simulink model "Prosthesis"  (R2014a)
settings: Solver=ode15s  StartTime=0.0  StopTime=20  MaxStep=.01  RelTol=1e-4  AbsTol=1e-5
InitFcn:
  | RphiKnee0 = 0*pi/180;
  | RphiAnkle0 = 0;
  | prostheticParams
StartFcn:
  | tic;
StopFcn:
  | toc
values from neighbouring files (symbols this model uses):
  ankleBackDriveGain = 0.8    [prostheticParams.m]
  ankleDgain = 0.001    [prostheticParams.m]
  ankleFilterPID = 100    [prostheticParams.m]
  ankleFilterSEA = 100    [prostheticParams.m]
  ankleGearEff = 1.00    (= 1)    [prostheticParams.m]
  ankleGearRatio = 50    [prostheticParams.m]
  ankleIgain = 0.00    (= 0)    [prostheticParams.m]
  ankleInitialAngle = -RphiAnkle0    [prostheticParams.m]
  ankleInputMass = 2329.69    [prostheticParams.m]
  ankleParallelSpringDamping = ankleParallelSpringStiffness/200    (= 0.95)    [prostheticParams.m]
  ankleParallelSpringOffset = 0    [prostheticParams.m]
  ankleParallelSpringStiffness = 190    [prostheticParams.m]
  anklePgain = 0.01    [prostheticParams.m]
  ankleSEADamping = ankleSEAStiffness/100    (= 15)    [prostheticParams.m]
  ankleSEAStiffness = 1500    [prostheticParams.m]
  ankleTendonMass = 36.26    [prostheticParams.m]
  footMassp = 690.10    (= 690.1)    [prostheticParams.m]
  FourBarL1 = 0.080    (= 0.08)    [prostheticParams.m]
  FourBarL3 = 0.0826238    [prostheticParams.m]
  kneeBackDriveGain = 0.8    [prostheticParams.m]
  kneeDgain = 0.001    [prostheticParams.m]
  kneeFilterPID = 100    [prostheticParams.m]
  kneeFilterSEA = 100    [prostheticParams.m]
  kneeGearEff = 1.00    (= 1)    [prostheticParams.m]
  kneeGearRatio = 50    [prostheticParams.m]
  kneeIgain = 0.00    (= 0)    [prostheticParams.m]
  kneeInitialAngle = -RphiKnee0    [prostheticParams.m]
  kneePgain = 0.01    [prostheticParams.m]
  kneeSEADamping = kneeSEAStiffness/100    (= 15)    [prostheticParams.m]
  kneeSEAStiffness = 1500    [prostheticParams.m]
  kneeStatorMass = 1519.39    [prostheticParams.m]
  motorBackEMF = 0.09167    [prostheticParams.m]
  motorInductance = 120e-6    (= 0.00012)    [prostheticParams.m]
  motorMaxCurrent = 4.5/motorTorsionalConst    (= 34.6153846154)    [prostheticParams.m]
  motorMaxVoltage = 48    [prostheticParams.m]
  motorResistance = .055    (= 0.055)    [prostheticParams.m]
  motorRotorInertia = motorRotorMomentOfInertia(3)*gcm2TOkgm2    [prostheticParams.m]
  motorRotorMass = 365.43    [prostheticParams.m]
  motorTorsionalConst = 0.130    (= 0.13)    [prostheticParams.m]
  shankMassp = 2329.69    [prostheticParams.m]
undefined symbols (not defined in the file or in its folder): X, Y, Z
undefined symbols (not defined in the file): ankleIntCoulomb, ankleIntDamping, ankleIntStatic, dryFrictionDamping, dryFrictionStiffness, dryFrictionVelThresh, kneeCJointstop, kneeExtCoulomb, kneeExtDamping, kneeExtStatic, kneeIntCoulomb, kneeIntDamping, kneeIntStatic, kneeWMaxJointstop
libraries: sm_lib x41, nesl_utility x16, simulink x4, NeuroMuscularLibrary x1
(part 1 of 2)
settings Model: Creator=nitisht  LastModifiedBy=nitisht
settings SolverCC: MaxConsecutiveZCs=100  ZeroCrossAlgorithm=Adaptive
settings OptimizationCC: AccelVerboseBuild=on
settings DebuggingCC: UnderspecifiedInitializationDetection=Classic  StateNameClashWarn=warning

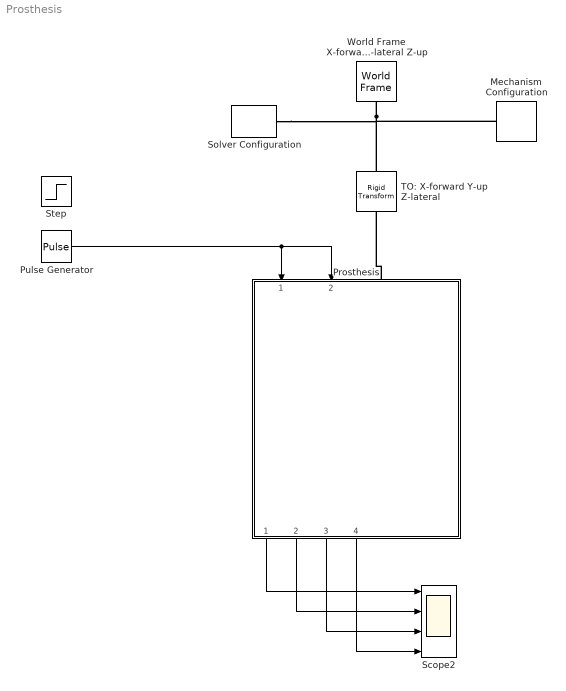
== system Prosthesis ==
  Mechanism Configuration : sm_lib/Utilities/Mechanism Configuration  UniformGravity=Constant  GravityVector=[0 0 -9.81]  GravityUnits=m/s^2  LinearizationDelta=0.001  BlockFunction=simmechanics.library.utilities.mechanism_configuration
  Prosthesis : Subsystem  AncestorBlock=NeuroMuscularLibrary/Full Prosthesis
  Pulse Generator : DiscretePulseGenerator  PulseType=Time based  Amplitude=50  Period=4  PulseWidth=50
  Scope2 : Scope  NumInputPorts=4
      settings: TimeRange=1  YMin=-1.5~-5~-12~-5  YMax=3.25~5~11~5  SaveName=ScopeData2
  Solver Configuration : nesl_utility/Solver Configuration  PhysicalDomain=network_engine_domain  SubClassName=solver  LeftPortType=input  RightPortType=generic  Accelerate=off  Tones=[]  Harmonics=[]  SimulateNoise=off  Profile=off  UseLocalSampling=off  EnableSwitchedLinearOptims=on  FrequencyDomain=off  UseCCode=off  RelTol=0.001  AbsTol=1e-06  MinStep=1e-09  ToWorkspace=off  DoDC=off  ResidualTolerance=1e-09  UseLocalSolver=off  LocalSolverChoice=NE_BACKWARD_EULER_ADVANCER  LocalSolverSampleTime=0.001  DoFixedCost=off  MaxNonlinIter=3  MaxModeIter=2  LinearAlgebra=Sparse  DelaysMemoryBudget=1024  AutomaticFiltering=on  FilteringTimeConstant=0.001
  Step : Step  Time=0  After=0  SampleTime=0
  TO: X-forward Y-up Z-lateral : sm_lib/Frames and Transforms/Rigid Transform  TranslationMethod=None  TranslationLengthUnit=m  TranslationStandardAxis=+Z  TranslationStandardOffset=0  TranslationCartesianOffset=[0 0 0]  TranslationROffset=0  TranslationROffsetUnits=m  TranslationZOffset=0  TranslationZOffsetUnits=m  TranslationThetaOffset=0  TranslationThetaOffsetUnits=deg  RotationMethod=AlignedAxes  RotationAngleUnits=deg  RotationStandardAxis=+Z  RotationAngle=0  RotationArbitraryAxis=[0 0 1]  FollAlignAxisA=+Y  BaseAlignAxisA=+Z  FollAlignAxisB=+X  BaseAlignAxisB=+X  BlockFunction=simmechanics.library.frames_transforms.rigid_transform
  World Frame X-forward Y-lateral Z-up : sm_lib/Frames and Transforms/World Frame  BlockFunction=simmechanics.library.frames_transforms.world_frame
  wires:
  Pulse Generator/1 -> Prosthesis/1(Desired Knee Torque), Prosthesis/2(Desired Ankle Torque)
  Prosthesis/1(Knee Angle) -> Scope2/1
  Prosthesis/2(Knee Speed) -> Scope2/2
  Prosthesis/3(Ankle Angle) -> Scope2/3
  Prosthesis/4(Ankle Speed) -> Scope2/4
  connections:
  World Frame X-forward Y-lateral Z-up/RConn1 -- Solver Configuration/RConn1 -- TO: X-forward Y-up Z-lateral/LConn1 -- Mechanism Configuration/RConn1
  Prosthesis/LConn1 -- TO: X-forward Y-up Z-lateral/RConn1

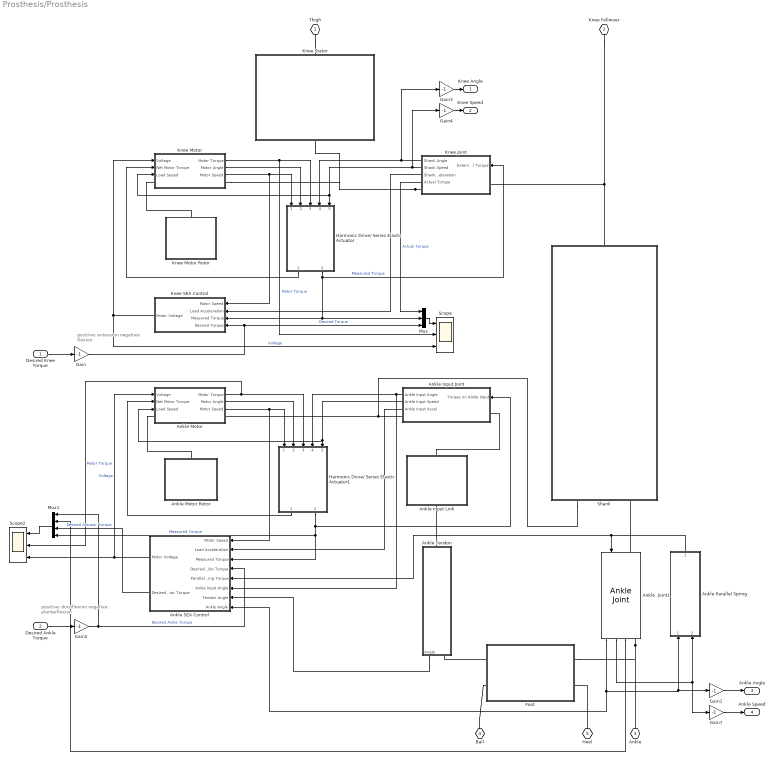
== system Prosthesis/Prosthesis ==
  note: positive: dorsiflexion
      | negative: plantarflexion
  note: positive: extension
      | negative: flexion
  Desired Knee Torque : Inport
  Desired Ankle Torque : Inport  Port=2
  Ankle  Joint1 : NeuroMuscularLibrary/Full Prosthesis No Motor/Ankle  Joint
      link override Ankle Joint: ClassName=RevoluteJoint  SenseConstraintForce=off  SenseConstraintForceX=off  SenseConstraintForceY=off  SenseConstraintForceZ=off  SenseConstraintTorque=off  SenseConstraintTorqueX=off  SenseConstraintTorqueY=off  SenseConstraintTorqueZ=off  SenseTotalForce=off  SenseTotalForceX=off  SenseTotalForceY=off  SenseTotalForceZ=off  SenseTotalTorque=off  SenseTotalTorqueX=off  SenseTotalTorqueY=off  SenseTotalTorqueZ=off  CompositeWrenchDir=FollowerOnBase  CompositeWrenchFrame=BaseFrame  EquilibriumPosition=0  EquilibriumPositionUnits=deg  SpringStiffness=100  SpringStiffnessUnits=N*m/rad  DampingCoefficient=10  DampingCoefficientUnits=N*m/(rad/s)  TorqueActuationMode=InputTorque  MotionActuationMode=ComputedMotion  SensePosition=on  SenseVelocity=on  SenseAcceleration=off  SenseTorqueForce=off  PositionTargetValue=0  PositionTargetValueUnits=rad  PositionTargetSpecify=on  PositionTargetPriority=Low  VelocityTargetValue=0  VelocityTargetValueUnits=deg/s  VelocityTargetSpecify=off  VelocityTargetPriority=High  BlockFunction=simmechanics.library.joints.revolute_joint
  Ankle Input Joint : Subsystem
  Ankle Input Link : Subsystem
      mask Display: image('ankleInputLinkThumb.png')
  Ankle Motor : Subsystem
  Ankle Motor Rotor : Subsystem
      mask Display: image('motorRotorThumb.png')
  Ankle Parallel Spring : Subsystem
  Ankle SEA Control : Subsystem
  Ankle Tendon : Subsystem
      mask Display: image('ankleTendonThumb.png')
  Foot : Subsystem
      mask Display: image('footThumb.png')
  Gain{,1..4,7} (6 alike) : Gain  Gain=-1
  Harmonic Drive/ Series Elastic Actuator : Subsystem
  Harmonic Drive/ Series Elastic Actuator1 : Subsystem
  Knee Joint : Subsystem
  Knee Motor : Subsystem
  Knee Motor Rotor : Subsystem
      mask Display: image('motorRotorThumb.png')
  Knee SEA Control : Subsystem
  Knee Stator : Subsystem
      mask Display: image('kneeStatorThumb.png')
  Mux : Mux  Inputs=3
  Mux1 : Mux
  Scope : Scope  NumInputPorts=3
      settings: ShowLegends=on  TimeRange=20  YMin=-100~-4.5~-50  YMax=50~4.5~50
  Scope2 : Scope  NumInputPorts=3
      settings: ShowLegends=on  TimeRange=1  YMin=-140~-4.5~-25  YMax=90~4.5~50
  Shank : Subsystem
      mask Display: image('shankThumb.png')
  Thigh : PMIOPort  Port=1  Side=Left
  Knee Follwoer : PMIOPort  Port=2  Side=Left
  Ankle : PMIOPort  Port=3  Side=Right
  Ball : PMIOPort  Port=4  Side=Right
  Heel : PMIOPort  Port=5  Side=Right
  Knee Angle : Outport
  Knee Speed : Outport  Port=2
  Ankle Angle : Outport  Port=3
  Ankle Speed : Outport  Port=4
  wires:
  Ankle  Joint1/3 -> Mux1/2
  Ankle  Joint1/2 -> Gain7/1, Ankle Parallel Spring/2(Ankle Speed)
  Ankle  Joint1/1 -> Ankle SEA Control/8(Ankle Angle), Gain1/1, Ankle Parallel Spring/1(Ankle Angle)
  Gain4/1 -> Knee Speed/1
  Gain3/1 -> Knee Angle/1
  Desired Ankle Torque/1 -> Gain2/1
  Desired Knee Torque/1 -> Gain/1
  Ankle Parallel Spring/1(Parallel Spring Torque) -> Ankle SEA Control/5(Parallel Spring Torque), Ankle  Joint1/1
  Harmonic Drive/ Series Elastic Actuator/2(" Torque on Load") -> Knee Joint/1(External Torque), Mux/2, Knee SEA Control/3(Measured Torque)  "Measured Torque"
  Gain/1 -> Knee SEA Control/4(Desired Torque), Mux/3  "Desired Torque"
  Mux/1 -> Scope/1
  Ankle Input Joint/2(Ankle Input Speed) -> Harmonic Drive/ Series Elastic Actuator1/5(Load Speed), Ankle Motor/3(Load Speed)
  Ankle Tendon/1(Angle) -> Ankle SEA Control/7(Tendon Angle)
  Ankle Input Joint/3(Ankle Input Accel) -> Ankle SEA Control/2(Load Acceleration)
  Harmonic Drive/ Series Elastic Actuator1/1(Torque on Motor) -> Ankle Motor/2(Net Motor Torque)
  Ankle Input Joint/1(Ankle Input Angle) -> Harmonic Drive/ Series Elastic Actuator1/4(Load Angle), Ankle SEA Control/6(Ankle Input Angle)
  Ankle Motor/3(Motor Speed) -> Harmonic Drive/ Series Elastic Actuator1/1(Motor Speed), Ankle SEA Control/1(Motor Speed)
  Ankle Motor/2(Motor Angle) -> Harmonic Drive/ Series Elastic Actuator1/2(Motor Angle)
  Knee Joint/3(Shank Acceleration) -> Knee SEA Control/2(Load Acceleration)
  Knee SEA Control/1(Motor Voltage) -> Knee Motor/1(Voltage), Scope/3  "Voltage"
  Knee Joint/2(Shank Speed) -> Harmonic Drive/ Series Elastic Actuator/5(Load Speed), Knee Motor/3(Load Speed), Gain4/1
  Knee Joint/1(Shank Angle) -> Harmonic Drive/ Series Elastic Actuator/4(Load Angle), Gain3/1
  Harmonic Drive/ Series Elastic Actuator/1(Torque on Motor) -> Knee Motor/2(Net Motor Torque)
  Knee Motor/1(Motor Torque) -> Scope/2, Harmonic Drive/ Series Elastic Actuator/3(Motor Torque)  "Motor Torque"
  Knee Motor/3(Motor Speed) -> Knee SEA Control/1(Motor Speed), Harmonic Drive/ Series Elastic Actuator/1(Motor Speed)
  Knee Motor/2(Motor Angle) -> Harmonic Drive/ Series Elastic Actuator/2(Motor Angle)
  Knee Joint/4(Actual Torque) -> Mux/1  "Actual Torque"
  Gain1/1 -> Ankle Angle/1
  Gain7/1 -> Ankle Speed/1
  Ankle SEA Control/1(Motor Voltage) -> Scope2/3, Ankle Motor/1(Voltage)  "Voltage"
  Ankle Motor/1(Motor Torque) -> Scope2/2, Harmonic Drive/ Series Elastic Actuator1/3(Motor Torque)  "Motor Torque"
  Harmonic Drive/ Series Elastic Actuator1/2(Torque on Load) -> Ankle SEA Control/3(Measured Torque), Mux1/4, Ankle Input Joint/1(Torque on Ankle Input)  "Measured Torque"
  Gain2/1 -> Mux1/1, Ankle SEA Control/4(Desired Ankle Torque)  "Desired Ankle Torque"
  Mux1/1 -> Scope2/1
  Ankle SEA Control/2(Desired Actuator Torque) -> Mux1/3  "Desired Actuaor Torque"
  connections:
  Heel/RConn1 -- Foot/RConn2
  Ball/RConn1 -- Foot/LConn2
  Foot/LConn1 -- Ankle Tendon/RConn1
  Ankle Tendon/LConn1 -- Ankle Input Link/LConn1
  Ankle  Joint1/RConn1 -- Ankle/RConn1 -- Foot/RConn1
  Ankle  Joint1/LConn1 -- Shank/LConn2
  Ankle Input Link/RConn1 -- Ankle Input Joint/LConn1
  Ankle Motor Rotor/RConn1 -- Ankle Motor/LConn1
  Ankle Input Joint/RConn1 -- Ankle Motor/RConn1 -- Shank/LConn1
  Knee Follwoer/RConn1 -- Knee Joint/LConn1 -- Shank/RConn1
  Knee Motor Rotor/RConn1 -- Knee Motor/LConn1
  Knee Joint/RConn1 -- Knee Motor/RConn1 -- Knee Stator/LConn1
  Thigh/RConn1 -- Knee Stator/RConn1

== system Prosthesis/Prosthesis/Ankle Input Joint ==
  Torque on Ankle Input : Inport
  Ankle Input Joint : sm_lib/Joints/Revolute Joint  SenseConstraintForce=off  SenseConstraintForceX=off  SenseConstraintForceY=off  SenseConstraintForceZ=off  SenseConstraintTorque=off  SenseConstraintTorqueX=off  SenseConstraintTorqueY=off  SenseConstraintTorqueZ=off  SenseTotalForce=off  SenseTotalForceX=off  SenseTotalForceY=off  SenseTotalForceZ=off  SenseTotalTorque=off  SenseTotalTorqueX=off  SenseTotalTorqueY=off  SenseTotalTorqueZ=off  CompositeWrenchDir=FollowerOnBase  CompositeWrenchFrame=BaseFrame  EquilibriumPosition=0  EquilibriumPositionUnits=rad  SpringStiffness=0  SpringStiffnessUnits=N*m/deg  DampingCoefficient=0  DampingCoefficientUnits=N*m/(deg/s)  TorqueActuationMode=InputTorque  MotionActuationMode=ComputedMotion  SensePosition=on  SenseVelocity=on  SenseAcceleration=on  SenseTorqueForce=off  PositionTargetValue=ankleInitialAngle  PositionTargetValueUnits=rad  PositionTargetSpecify=on  PositionTargetPriority=High  VelocityTargetValue=0  VelocityTargetValueUnits=deg/s  VelocityTargetSpecify=off  VelocityTargetPriority=High  BlockFunction=simmechanics.library.joints.revolute_joint
  PS-Simulink Converter1 : nesl_utility/PS-Simulink Converter  PhysicalDomain=network_engine_domain  SubClassName=ps_output  LeftPortType=input  RightPortType=output  PseudoPeriodic=off  Frequencies=[]  Unit=rad/s^2  AffineConversion=off
  PS-Simulink Converter2 : nesl_utility/PS-Simulink Converter  PhysicalDomain=network_engine_domain  SubClassName=ps_output  LeftPortType=input  RightPortType=output  PseudoPeriodic=off  Frequencies=[]  Unit=rad  AffineConversion=off
  PS-Simulink Converter3 : nesl_utility/PS-Simulink Converter  PhysicalDomain=network_engine_domain  SubClassName=ps_output  LeftPortType=input  RightPortType=output  PseudoPeriodic=off  Frequencies=[]  Unit=rad/s  AffineConversion=off
  Rigid Transform : sm_lib/Frames and Transforms/Rigid Transform  TranslationMethod=None  TranslationLengthUnit=m  TranslationStandardAxis=+Z  TranslationStandardOffset=0  TranslationCartesianOffset=[0 0 0]  TranslationROffset=0  TranslationROffsetUnits=m  TranslationZOffset=0  TranslationZOffsetUnits=m  TranslationThetaOffset=0  TranslationThetaOffsetUnits=deg  RotationMethod=StandardAxis  RotationAngleUnits=deg  RotationStandardAxis=+Z  RotationAngle=180  RotationArbitraryAxis=[0 0 1]  FollAlignAxisA=+X  BaseAlignAxisA=+Y  FollAlignAxisB=+Y  BaseAlignAxisB=+Z  BlockFunction=simmechanics.library.frames_transforms.rigid_transform
  Simulink-PS Converter : nesl_utility/Simulink-PS Converter  PhysicalDomain=network_engine_domain  SubClassName=ps_input  LeftPortType=input  RightPortType=output  PseudoPeriodic=off  Frequencies=[]  NoiseDistribution=none  NoiseParameters=[]  Unit=N*m  AffineConversion=off  InputFiltering=off  SimscapeFilterOrder=1  InputFilterTimeConstant=0.001  UdotUserProvided=1
  Ankle Stator : PMIOPort  Port=1  Side=Right
  Ankle Input : PMIOPort  Port=2  Side=Left
  Ankle Input Angle : Outport
  Ankle Input Speed : Outport  Port=2
  Ankle Input Accel : Outport  Port=3
  wires:
  Torque on Ankle Input/1 -> Simulink-PS Converter/1
  PS-Simulink Converter1/1 -> Ankle Input Accel/1
  PS-Simulink Converter3/1 -> Ankle Input Speed/1
  PS-Simulink Converter2/1 -> Ankle Input Angle/1
  connections:
  Rigid Transform/LConn1 -- Ankle Stator/RConn1
  Ankle Input Joint/LConn1 -- Rigid Transform/RConn1
  Ankle Input Joint/RConn4 -- PS-Simulink Converter1/LConn1
  Ankle Input Joint/LConn2 -- Simulink-PS Converter/RConn1
  Ankle Input Joint/RConn2 -- PS-Simulink Converter2/LConn1
  Ankle Input Joint/RConn3 -- PS-Simulink Converter3/LConn1
  Ankle Input Joint/RConn1 -- Ankle Input/RConn1

== system Prosthesis/Prosthesis/Ankle Input Link ==
  CG : sm_lib/Frames and Transforms/Reference Frame  BlockFunction=simmechanics.library.frames_transforms.reference_frame
  Shank : sm_lib/Body Elements/Solid  InertiaType=Custom  Mass=ankleInputMass  MassUnits=g  CenterOfMass=ankleInputCG  CenterOfMassUnits=mm  MomentsOfInertia=ankleInputMomentOfInertia  MomentsOfInertiaUnits=g*cm^2  ProductsOfInertia=ankleInputProductOfInertia  ProductsOfInertiaUnits=g*cm^2  DensityBased=on  Density=1000  DensityUnits=kg/(m^3)  GraphicType=FromGeometry  MarkerShape=Sphere  MarkerSize=10  MarkerSizeUnits=m  GraphicVisPropType=SimpleVisualProperties  GraphicDiffuseColor=[0.5 0.5 0.5]  GraphicSpecularColor=[0.5 0.5 0.5 1.0]  GraphicAmbientColor=[0.15 0.15 0.15 1.0]  GraphicEmissiveColor=[0.0 0.0 0.0 1.0]  GraphicShininess=75  GraphicOpacity=1.0  GeometryShape=FromFile  RectangleSize=[1 1]  RectangleSizeUnits=m  BrickDimensions=[1 1 1]  BrickDimensionUnits=m  CylinderRadius=1  CylinderRadiusUnits=m  CylinderLength=1  CylinderLengthUnits=m  SphereRadius=1  SphereRadiusUnits=m  EllipsoidRadii=[1 1 1]  EllipsoidRadiiUnits=m  ExtrusionCrossSection=[1 1; -1 1; -1 -1; 1 -1]  ExtrusionCrossSectionUnits=m  ExtrusionLength=1  ExtrusionLengthUnits=m  PolygonNumSides=3  PolygonOuterRadius=1  PolygonOuterRadiusUnits=m  ExtGeomFileType=STL  ExtGeomFileName=ankleInputLink.STL  ExtGeomFileUnits=mm  RevolutionCrossSection=[1 1; 1 -1; 2 -1; 2 1]  RevolutionCrossSectionUnits=m  RevolutionExtent=Full  RevolutionAngle=180  RevolutionAngleUnits=deg  BlockFunction=simmechanics.library.body_elements.solid
  To CG : sm_lib/Frames and Transforms/Rigid Transform  TranslationMethod=Cartesian  TranslationLengthUnit=mm  TranslationStandardAxis=-Z  TranslationStandardOffset=1.5  TranslationCartesianOffset=ankleInputCG  TranslationROffset=0  TranslationROffsetUnits=m  TranslationZOffset=0  TranslationZOffsetUnits=m  TranslationThetaOffset=0  TranslationThetaOffsetUnits=deg  RotationMethod=None  RotationAngleUnits=deg  RotationStandardAxis=+Z  RotationAngle=0  RotationArbitraryAxis=[0 0 1]  FollAlignAxisA=+X  BaseAlignAxisA=+Y  FollAlignAxisB=+Y  BaseAlignAxisB=+Z  BlockFunction=simmechanics.library.frames_transforms.rigid_transform
  To Tendon : sm_lib/Frames and Transforms/Rigid Transform  TranslationMethod=Cartesian  TranslationLengthUnit=mm  TranslationStandardAxis=-Y  TranslationStandardOffset=445.61  TranslationCartesianOffset=[80, 0, 2]  TranslationROffset=0  TranslationROffsetUnits=m  TranslationZOffset=0  TranslationZOffsetUnits=m  TranslationThetaOffset=0  TranslationThetaOffsetUnits=deg  RotationMethod=None  RotationAngleUnits=deg  RotationStandardAxis=+Z  RotationAngle=0  RotationArbitraryAxis=[0 0 1]  FollAlignAxisA=+X  BaseAlignAxisA=+Y  FollAlignAxisB=+Y  BaseAlignAxisB=+Z  BlockFunction=simmechanics.library.frames_transforms.rigid_transform
  " Ankle Input Joint" : PMIOPort  Port=1  Side=Right
  Tendon : PMIOPort  Port=2  Side=Left
  connections:
  Shank/RConn1 -- To CG/LConn1 -- " Ankle Input Joint"/RConn1 -- To Tendon/LConn1
  CG/RConn1 -- To CG/RConn1
  Tendon/RConn1 -- To Tendon/RConn1

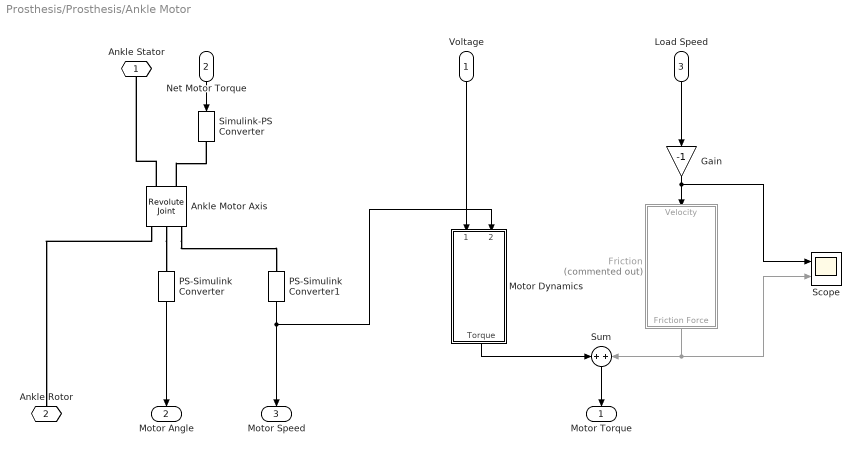
== system Prosthesis/Prosthesis/Ankle Motor ==
  Voltage : Inport
  Net Motor Torque : Inport  Port=2
  Load Speed : Inport  Port=3
  Ankle Motor Axis : sm_lib/Joints/Revolute Joint  SenseConstraintForce=off  SenseConstraintForceX=off  SenseConstraintForceY=off  SenseConstraintForceZ=off  SenseConstraintTorque=off  SenseConstraintTorqueX=off  SenseConstraintTorqueY=off  SenseConstraintTorqueZ=off  SenseTotalForce=off  SenseTotalForceX=off  SenseTotalForceY=off  SenseTotalForceZ=off  SenseTotalTorque=off  SenseTotalTorqueX=off  SenseTotalTorqueY=off  SenseTotalTorqueZ=off  CompositeWrenchDir=FollowerOnBase  CompositeWrenchFrame=BaseFrame  EquilibriumPosition=0  EquilibriumPositionUnits=deg  SpringStiffness=0  SpringStiffnessUnits=N*m/deg  DampingCoefficient=0  DampingCoefficientUnits=N*m/(deg/s)  TorqueActuationMode=InputTorque  MotionActuationMode=ComputedMotion  SensePosition=on  SenseVelocity=on  SenseAcceleration=off  SenseTorqueForce=off  PositionTargetValue=-ankleInitialAngle*ankleGearRatio  PositionTargetValueUnits=rad  PositionTargetSpecify=on  PositionTargetPriority=High  VelocityTargetValue=0  VelocityTargetValueUnits=deg/s  VelocityTargetSpecify=off  VelocityTargetPriority=High  BlockFunction=simmechanics.library.joints.revolute_joint
  Friction : Subsystem  Commented=on  mask{Fs=ankleIntStatic, Fc=ankleIntCoulomb, sigma0=dryFrictionStiffness, sigma1=dryFrictionDamping, v_s=dryFrictionVelThresh, Fv=ankleIntDamping}
      mask prompts: Fs "Static Friction"; Fc "Colulomb Friction"; sigma0 "Dry Friction Stiffness"; sigma1 "Dry Friction Damping"; v_s "Velocity Threshold"; Fv "Viscous Friction"
  Gain : Gain  Gain=-1
  Motor Dynamics : Subsystem
  PS-Simulink Converter : nesl_utility/PS-Simulink Converter  PhysicalDomain=network_engine_domain  SubClassName=ps_output  LeftPortType=input  RightPortType=output  PseudoPeriodic=off  Frequencies=[]  Unit=rad  AffineConversion=off
  PS-Simulink Converter1 : nesl_utility/PS-Simulink Converter  PhysicalDomain=network_engine_domain  SubClassName=ps_output  LeftPortType=input  RightPortType=output  PseudoPeriodic=off  Frequencies=[]  Unit=rad/s  AffineConversion=off
  Scope : Scope  NumInputPorts=2
      settings: TimeRange=3.5  YMin=-3.5~-0.25  YMax=1.5~0.15
  Simulink-PS Converter : nesl_utility/Simulink-PS Converter  PhysicalDomain=network_engine_domain  SubClassName=ps_input  LeftPortType=input  RightPortType=output  PseudoPeriodic=off  Frequencies=[]  NoiseDistribution=none  NoiseParameters=[]  Unit=N*m  AffineConversion=off  InputFiltering=off  SimscapeFilterOrder=1  InputFilterTimeConstant=0.001  UdotUserProvided=1
  Sum : Sum  Inputs=+|+
  Ankle Stator : PMIOPort  Port=1  Side=Right
  Ankle Rotor : PMIOPort  Port=2  Side=Left
  Motor Torque : Outport
  Motor Angle : Outport  Port=2
  Motor Speed : Outport  Port=3
  wires:
  Gain/1 -> Scope/1, Friction/1(Velocity)
  Load Speed/1 -> Gain/1
  Sum/1 -> Motor Torque/1
  Motor Dynamics/1(Torque) -> Sum/1
  PS-Simulink Converter1/1 -> Motor Speed/1, Motor Dynamics/2(Speed)
  Net Motor Torque/1 -> Simulink-PS Converter/1
  PS-Simulink Converter/1 -> Motor Angle/1
  Voltage/1 -> Motor Dynamics/1(Voltage)
  Friction/1(Friction Force) -> Scope/2, Sum/2
  connections:
  Ankle Motor Axis/RConn1 -- Ankle Rotor/RConn1
  Ankle Motor Axis/LConn2 -- Simulink-PS Converter/RConn1
  Ankle Motor Axis/RConn3 -- PS-Simulink Converter1/LConn1
  Ankle Motor Axis/RConn2 -- PS-Simulink Converter/LConn1
  Ankle Motor Axis/LConn1 -- Ankle Stator/RConn1

== system Prosthesis/Prosthesis/Ankle Motor Rotor ==
  CG : sm_lib/Frames and Transforms/Reference Frame  BlockFunction=simmechanics.library.frames_transforms.reference_frame
  Knee Rotor1 : sm_lib/Body Elements/Solid  InertiaType=Custom  Mass=motorRotorMass  MassUnits=g  CenterOfMass=motorRotorCG  CenterOfMassUnits=mm  MomentsOfInertia=motorRotorMomentOfInertia  MomentsOfInertiaUnits=g*cm^2  ProductsOfInertia=motorRotorProductOfInertia  ProductsOfInertiaUnits=g*cm^2  DensityBased=on  Density=1000  DensityUnits=kg/(m^3)  GraphicType=FromGeometry  MarkerShape=Sphere  MarkerSize=10  MarkerSizeUnits=m  GraphicVisPropType=SimpleVisualProperties  GraphicDiffuseColor=[0.5 0.5 0.5]  GraphicSpecularColor=[0.5 0.5 0.5 1.0]  GraphicAmbientColor=[0.15 0.15 0.15 1.0]  GraphicEmissiveColor=[0.0 0.0 0.0 1.0]  GraphicShininess=75  GraphicOpacity=1.0  GeometryShape=FromFile  RectangleSize=[1 1]  RectangleSizeUnits=m  BrickDimensions=[1 1 1]  BrickDimensionUnits=m  CylinderRadius=1  CylinderRadiusUnits=m  CylinderLength=1  CylinderLengthUnits=m  SphereRadius=1  SphereRadiusUnits=m  EllipsoidRadii=[1 1 1]  EllipsoidRadiiUnits=m  ExtrusionCrossSection=[1 1; -1 1; -1 -1; 1 -1]  ExtrusionCrossSectionUnits=m  ExtrusionLength=1  ExtrusionLengthUnits=m  PolygonNumSides=3  PolygonOuterRadius=1  PolygonOuterRadiusUnits=m  ExtGeomFileType=STL  ExtGeomFileName=motorRotor.STL  ExtGeomFileUnits=mm  RevolutionCrossSection=[1 1; 1 -1; 2 -1; 2 1]  RevolutionCrossSectionUnits=m  RevolutionExtent=Full  RevolutionAngle=180  RevolutionAngleUnits=deg  BlockFunction=simmechanics.library.body_elements.solid
  Rigid Transform : sm_lib/Frames and Transforms/Rigid Transform  TranslationMethod=StandardAxis  TranslationLengthUnit=mm  TranslationStandardAxis=+Z  TranslationStandardOffset=4.5  TranslationCartesianOffset=[0 0 0]  TranslationROffset=0  TranslationROffsetUnits=m  TranslationZOffset=0  TranslationZOffsetUnits=m  TranslationThetaOffset=0  TranslationThetaOffsetUnits=deg  RotationMethod=None  RotationAngleUnits=deg  RotationStandardAxis=+Z  RotationAngle=0  RotationArbitraryAxis=[0 0 1]  FollAlignAxisA=+X  BaseAlignAxisA=+Y  FollAlignAxisB=+Y  BaseAlignAxisB=+Z  BlockFunction=simmechanics.library.frames_transforms.rigid_transform
  ToCG : sm_lib/Frames and Transforms/Rigid Transform  TranslationMethod=Cartesian  TranslationLengthUnit=mm  TranslationStandardAxis=+Z  TranslationStandardOffset=0  TranslationCartesianOffset=motorRotorCG  TranslationROffset=0  TranslationROffsetUnits=m  TranslationZOffset=0  TranslationZOffsetUnits=m  TranslationThetaOffset=0  TranslationThetaOffsetUnits=deg  RotationMethod=None  RotationAngleUnits=deg  RotationStandardAxis=+Z  RotationAngle=0  RotationArbitraryAxis=[0 0 1]  FollAlignAxisA=+X  BaseAlignAxisA=+Y  FollAlignAxisB=+Y  BaseAlignAxisB=+Z  BlockFunction=simmechanics.library.frames_transforms.rigid_transform
  Conn1 : PMIOPort  Port=1  Side=Right
  connections:
  Conn1/RConn1 -- Rigid Transform/LConn1
  Rigid Transform/RConn1 -- Knee Rotor1/RConn1 -- ToCG/LConn1
  CG/RConn1 -- ToCG/RConn1

== system Prosthesis/Prosthesis/Ankle Parallel Spring ==
  Ankle Angle : Inport
  Ankle Speed : Inport  Port=2
  Add : Sum
  Bias : Bias  Bias=-ankleParallelSpringOffset
  Parallel Spring Stiffness : Gain  Gain=-ankleParallelSpringStiffness
  Parallel Spring Damping : Gain  Gain=-ankleParallelSpringDamping
  Saturation1 : Saturate  UpperLimit=0  LowerLimit=-inf  ZeroCross=off
  Saturation2 : Saturate  UpperLimit=0  LowerLimit=-inf  ZeroCross=off
  Parallel Spring Torque : Outport
  wires:
  Saturation2/1 -> Add/1
  Saturation1/1 -> Add/2
  Ankle Angle/1 -> Bias/1
  Bias/1 -> Parallel Spring Stiffness/1
  Parallel Spring Damping/1 -> Saturation1/1
  Parallel Spring Stiffness/1 -> Saturation2/1
  Ankle Speed/1 -> Parallel Spring Damping/1
  Add/1 -> Parallel Spring Torque/1

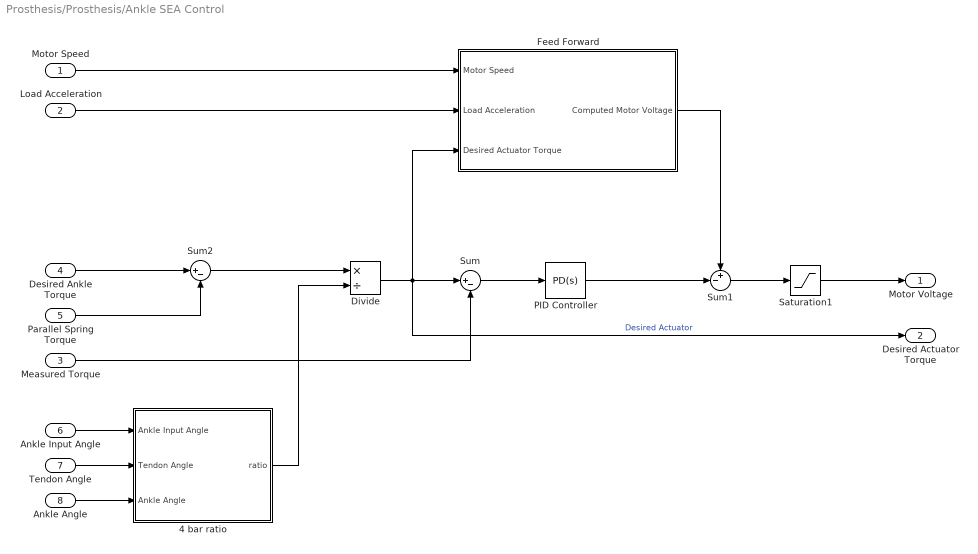
== system Prosthesis/Prosthesis/Ankle SEA Control ==
  Motor Speed : Inport
  Load Acceleration : Inport  Port=2
  Measured Torque : Inport  Port=3
  Desired Ankle Torque : Inport  Port=4
  Parallel Spring Torque : Inport  Port=5
  Ankle Input Angle : Inport  Port=6
  Tendon Angle : Inport  Port=7
  Ankle Angle : Inport  Port=8
  4 bar ratio : Subsystem
  Divide : Product  Inputs=*/
  Feed Forward : Subsystem
  PID Controller : simulink/Continuous/PID Controller  Controller=PD  TimeDomain=Continuous-time  SampleTime=.001  IntegratorMethod=Forward Euler  FilterMethod=Forward Euler  Form=Parallel  P=anklePgain  I=ankleIgain  D=ankleDgain  N=ankleFilterPID  InitialConditionSource=internal  InitialConditionForIntegrator=0  InitialConditionForFilter=0  ExternalReset=none  LimitOutput=off  UpperSaturationLimit=inf  LowerSaturationLimit=-inf  LinearizeAsGain=on  AntiWindupMode=none  Kb=1  TrackingMode=off  Kt=1  PParamMin=[]  PParamMax=[]  IParamMin=[]  IParamMax=[]  DParamMin=[]  DParamMax=[]  NParamMin=[]  NParamMax=[]  KbParamMin=[]  KbParamMax=[]  KtParamMin=[]  KtParamMax=[]  POutMin=[]  POutMax=[]  IOutMin=[]  IOutMax=[]  DOutMin=[]  DOutMax=[]  NOutMin=[]  NOutMax=[]  KbOutMin=[]  KbOutMax=[]  KtOutMin=[]  KtOutMax=[]  IntegratorOutMin=[]  IntegratorOutMax=[]  FilterOutMin=[]  FilterOutMax=[]  SumOutMin=[]  SumOutMax=[]  SumI1OutMin=[]  SumI1OutMax=[]  SumI2OutMin=[]  SumI2OutMax=[]  SumI3OutMin=[]  SumI3OutMax=[]  SumDOutMin=[]  SumDOutMax=[]  SaturationOutMin=[]  SaturationOutMax=[]  IntegratorContinuousStateAttributes=''  IntegratorStateMustResolveToSignalObject=off  IntegratorRTWStateStorageClass=Auto  FilterContinuousStateAttributes=''  FilterStateMustResolveToSignalObject=off  FilterRTWStateStorageClass=Auto
  Saturation1 : Saturate  UpperLimit=motorMaxVoltage  LowerLimit=-motorMaxVoltage  ZeroCross=off
  Sum : Sum  Inputs=|+-
  Sum1 : Sum  Inputs=+-|
  Sum2 : Sum  Inputs=|+-
  Motor Voltage : Outport
  Desired Actuator Torque : Outport  Port=2
  wires:
  PID Controller/1 -> Sum1/2
  Parallel Spring Torque/1 -> Sum2/2
  Desired Ankle Torque/1 -> Sum2/1
  Feed Forward/1(Computed Motor Voltage) -> Sum1/1
  Motor Speed/1 -> Feed Forward/1(Motor Speed)
  4 bar ratio/1(ratio) -> Divide/2
  Sum/1 -> PID Controller/1
  Measured Torque/1 -> Sum/2
  Ankle Angle/1 -> 4 bar ratio/3(Ankle Angle)
  Tendon Angle/1 -> 4 bar ratio/2(Tendon Angle)
  Ankle Input Angle/1 -> 4 bar ratio/1(Ankle Input Angle)
  Load Acceleration/1 -> Feed Forward/2(Load Acceleration)
  Sum1/1 -> Saturation1/1
  Saturation1/1 -> Motor Voltage/1
  Sum2/1 -> Divide/1
  Divide/1 -> Desired Actuator Torque/1, Feed Forward/3(Desired Actuator Torque), Sum/1  "Desired Actuator"

== system Prosthesis/Prosthesis/Ankle Tendon ==
  CG : sm_lib/Frames and Transforms/Reference Frame  BlockFunction=simmechanics.library.frames_transforms.reference_frame
  PS-Simulink Converter : nesl_utility/PS-Simulink Converter  PhysicalDomain=network_engine_domain  SubClassName=ps_output  LeftPortType=input  RightPortType=output  PseudoPeriodic=off  Frequencies=[]  Unit=1  AffineConversion=off
  Revolute Joint : sm_lib/Joints/Revolute Joint  SenseConstraintForce=off  SenseConstraintForceX=off  SenseConstraintForceY=off  SenseConstraintForceZ=off  SenseConstraintTorque=off  SenseConstraintTorqueX=off  SenseConstraintTorqueY=off  SenseConstraintTorqueZ=off  SenseTotalForce=off  SenseTotalForceX=off  SenseTotalForceY=off  SenseTotalForceZ=off  SenseTotalTorque=off  SenseTotalTorqueX=off  SenseTotalTorqueY=off  SenseTotalTorqueZ=off  CompositeWrenchDir=FollowerOnBase  CompositeWrenchFrame=BaseFrame  EquilibriumPosition=0  EquilibriumPositionUnits=deg  SpringStiffness=0  SpringStiffnessUnits=N*m/deg  DampingCoefficient=0  DampingCoefficientUnits=N*m/(deg/s)  TorqueActuationMode=NoTorque  MotionActuationMode=ComputedMotion  SensePosition=on  SenseVelocity=off  SenseAcceleration=off  SenseTorqueForce=off  PositionTargetValue=0  PositionTargetValueUnits=deg  PositionTargetSpecify=off  PositionTargetPriority=High  VelocityTargetValue=0  VelocityTargetValueUnits=deg/s  VelocityTargetSpecify=off  VelocityTargetPriority=High  BlockFunction=simmechanics.library.joints.revolute_joint
  Revolute Joint1 : sm_lib/Joints/Revolute Joint  SenseConstraintForce=off  SenseConstraintForceX=off  SenseConstraintForceY=off  SenseConstraintForceZ=off  SenseConstraintTorque=off  SenseConstraintTorqueX=off  SenseConstraintTorqueY=off  SenseConstraintTorqueZ=off  SenseTotalForce=off  SenseTotalForceX=off  SenseTotalForceY=off  SenseTotalForceZ=off  SenseTotalTorque=off  SenseTotalTorqueX=off  SenseTotalTorqueY=off  SenseTotalTorqueZ=off  CompositeWrenchDir=FollowerOnBase  CompositeWrenchFrame=BaseFrame  EquilibriumPosition=0  EquilibriumPositionUnits=deg  SpringStiffness=0  SpringStiffnessUnits=N*m/deg  DampingCoefficient=0  DampingCoefficientUnits=N*m/(deg/s)  TorqueActuationMode=NoTorque  MotionActuationMode=ComputedMotion  SensePosition=off  SenseVelocity=off  SenseAcceleration=off  SenseTorqueForce=off  PositionTargetValue=0  PositionTargetValueUnits=deg  PositionTargetSpecify=off  PositionTargetPriority=High  VelocityTargetValue=0  VelocityTargetValueUnits=deg/s  VelocityTargetSpecify=off  VelocityTargetPriority=High  BlockFunction=simmechanics.library.joints.revolute_joint
  Shank : sm_lib/Body Elements/Solid  InertiaType=Custom  Mass=ankleTendonMass  MassUnits=g  CenterOfMass=ankleTendonCG  CenterOfMassUnits=mm  MomentsOfInertia=ankleTendonMomentOfInertia  MomentsOfInertiaUnits=g*cm^2  ProductsOfInertia=ankleTendonProductOfInertia  ProductsOfInertiaUnits=g*cm^2  DensityBased=on  Density=1000  DensityUnits=kg/(m^3)  GraphicType=FromGeometry  MarkerShape=Sphere  MarkerSize=10  MarkerSizeUnits=m  GraphicVisPropType=SimpleVisualProperties  GraphicDiffuseColor=[0.5 0.5 0.5]  GraphicSpecularColor=[0.5 0.5 0.5 1.0]  GraphicAmbientColor=[0.15 0.15 0.15 1.0]  GraphicEmissiveColor=[0.0 0.0 0.0 1.0]  GraphicShininess=75  GraphicOpacity=1.0  GeometryShape=FromFile  RectangleSize=[1 1]  RectangleSizeUnits=m  BrickDimensions=[1 1 1]  BrickDimensionUnits=m  CylinderRadius=1  CylinderRadiusUnits=m  CylinderLength=1  CylinderLengthUnits=m  SphereRadius=1  SphereRadiusUnits=m  EllipsoidRadii=[1 1 1]  EllipsoidRadiiUnits=m  ExtrusionCrossSection=[1 1; -1 1; -1 -1; 1 -1]  ExtrusionCrossSectionUnits=m  ExtrusionLength=1  ExtrusionLengthUnits=m  PolygonNumSides=3  PolygonOuterRadius=1  PolygonOuterRadiusUnits=m  ExtGeomFileType=STL  ExtGeomFileName=ankleTendon.STL  ExtGeomFileUnits=mm  RevolutionCrossSection=[1 1; 1 -1; 2 -1; 2 1]  RevolutionCrossSectionUnits=m  RevolutionExtent=Full  RevolutionAngle=180  RevolutionAngleUnits=deg  BlockFunction=simmechanics.library.body_elements.solid
  To CG : sm_lib/Frames and Transforms/Rigid Transform  TranslationMethod=Cartesian  TranslationLengthUnit=mm  TranslationStandardAxis=-Z  TranslationStandardOffset=1.5  TranslationCartesianOffset=ankleTendonCG  TranslationROffset=0  TranslationROffsetUnits=m  TranslationZOffset=0  TranslationZOffsetUnits=m  TranslationThetaOffset=0  TranslationThetaOffsetUnits=deg  RotationMethod=None  RotationAngleUnits=deg  RotationStandardAxis=+Z  RotationAngle=0  RotationArbitraryAxis=[0 0 1]  FollAlignAxisA=+X  BaseAlignAxisA=+Y  FollAlignAxisB=+Y  BaseAlignAxisB=+Z  BlockFunction=simmechanics.library.frames_transforms.rigid_transform
  To Foot : sm_lib/Frames and Transforms/Rigid Transform  TranslationMethod=Cartesian  TranslationLengthUnit=mm  TranslationStandardAxis=-Y  TranslationStandardOffset=445.61  TranslationCartesianOffset=[0, -328.8, 0]  TranslationROffset=0  TranslationROffsetUnits=m  TranslationZOffset=0  TranslationZOffsetUnits=m  TranslationThetaOffset=0  TranslationThetaOffsetUnits=deg  RotationMethod=None  RotationAngleUnits=deg  RotationStandardAxis=+Z  RotationAngle=0  RotationArbitraryAxis=[0 0 1]  FollAlignAxisA=+X  BaseAlignAxisA=+Y  FollAlignAxisB=+Y  BaseAlignAxisB=+Z  BlockFunction=simmechanics.library.frames_transforms.rigid_transform
  " Ankle Input Joint" : PMIOPort  Port=1  Side=Left
  Foot : PMIOPort  Port=2  Side=Right
  Angle : Outport
  wires:
  PS-Simulink Converter/1 -> Angle/1
  connections:
  Revolute Joint/RConn2 -- PS-Simulink Converter/LConn1
  Foot/RConn1 -- Revolute Joint1/RConn1
  Revolute Joint1/LConn1 -- To Foot/RConn1
  Revolute Joint/LConn1 -- " Ankle Input Joint"/RConn1
  Shank/RConn1 -- To CG/LConn1 -- Revolute Joint/RConn1 -- To Foot/LConn1
  CG/RConn1 -- To CG/RConn1

== system Prosthesis/Prosthesis/Foot ==
  CG : sm_lib/Frames and Transforms/Reference Frame  BlockFunction=simmechanics.library.frames_transforms.reference_frame
  Shank : sm_lib/Body Elements/Solid  InertiaType=Custom  Mass=footMassp  MassUnits=g  CenterOfMass=footCG  CenterOfMassUnits=mm  MomentsOfInertia=footMomentOfInertia  MomentsOfInertiaUnits=g*cm^2  ProductsOfInertia=footProductOfInertia  ProductsOfInertiaUnits=g*cm^2  DensityBased=on  Density=1000  DensityUnits=kg/(m^3)  GraphicType=FromGeometry  MarkerShape=Sphere  MarkerSize=10  MarkerSizeUnits=m  GraphicVisPropType=SimpleVisualProperties  GraphicDiffuseColor=[0.5 0.5 0.5]  GraphicSpecularColor=[0.5 0.5 0.5 1.0]  GraphicAmbientColor=[0.15 0.15 0.15 1.0]  GraphicEmissiveColor=[0.0 0.0 0.0 1.0]  GraphicShininess=75  GraphicOpacity=1.0  GeometryShape=FromFile  RectangleSize=[1 1]  RectangleSizeUnits=m  BrickDimensions=[1 1 1]  BrickDimensionUnits=m  CylinderRadius=1  CylinderRadiusUnits=m  CylinderLength=1  CylinderLengthUnits=m  SphereRadius=1  SphereRadiusUnits=m  EllipsoidRadii=[1 1 1]  EllipsoidRadiiUnits=m  ExtrusionCrossSection=[1 1; -1 1; -1 -1; 1 -1]  ExtrusionCrossSectionUnits=m  ExtrusionLength=1  ExtrusionLengthUnits=m  PolygonNumSides=3  PolygonOuterRadius=1  PolygonOuterRadiusUnits=m  ExtGeomFileType=STL  ExtGeomFileName=foot.STL  ExtGeomFileUnits=mm  RevolutionCrossSection=[1 1; 1 -1; 2 -1; 2 1]  RevolutionCrossSectionUnits=m  RevolutionExtent=Full  RevolutionAngle=180  RevolutionAngleUnits=deg  BlockFunction=simmechanics.library.body_elements.solid
  To Ball : sm_lib/Frames and Transforms/Rigid Transform  TranslationMethod=Cartesian  TranslationLengthUnit=mm  TranslationStandardAxis=-Y  TranslationStandardOffset=445.61  TranslationCartesianOffset=[165, -63, 0]  TranslationROffset=0  TranslationROffsetUnits=m  TranslationZOffset=0  TranslationZOffsetUnits=m  TranslationThetaOffset=0  TranslationThetaOffsetUnits=deg  RotationMethod=None  RotationAngleUnits=deg  RotationStandardAxis=+Z  RotationAngle=0  RotationArbitraryAxis=[0 0 1]  FollAlignAxisA=+X  BaseAlignAxisA=+Y  FollAlignAxisB=+Y  BaseAlignAxisB=+Z  BlockFunction=simmechanics.library.frames_transforms.rigid_transform
  To CG : sm_lib/Frames and Transforms/Rigid Transform  TranslationMethod=Cartesian  TranslationLengthUnit=mm  TranslationStandardAxis=-Z  TranslationStandardOffset=1.5  TranslationCartesianOffset=footCG  TranslationROffset=0  TranslationROffsetUnits=m  TranslationZOffset=0  TranslationZOffsetUnits=m  TranslationThetaOffset=0  TranslationThetaOffsetUnits=deg  RotationMethod=None  RotationAngleUnits=deg  RotationStandardAxis=+Z  RotationAngle=0  RotationArbitraryAxis=[0 0 1]  FollAlignAxisA=+X  BaseAlignAxisA=+Y  FollAlignAxisB=+Y  BaseAlignAxisB=+Z  BlockFunction=simmechanics.library.frames_transforms.rigid_transform
  To Heel : sm_lib/Frames and Transforms/Rigid Transform  TranslationMethod=Cartesian  TranslationLengthUnit=mm  TranslationStandardAxis=-Y  TranslationStandardOffset=445.61  TranslationCartesianOffset=[-60, -63, 0]  TranslationROffset=0  TranslationROffsetUnits=m  TranslationZOffset=0  TranslationZOffsetUnits=m  TranslationThetaOffset=0  TranslationThetaOffsetUnits=deg  RotationMethod=None  RotationAngleUnits=deg  RotationStandardAxis=+Z  RotationAngle=0  RotationArbitraryAxis=[0 0 1]  FollAlignAxisA=+X  BaseAlignAxisA=+Y  FollAlignAxisB=+Y  BaseAlignAxisB=+Z  BlockFunction=simmechanics.library.frames_transforms.rigid_transform
  To Tendon : sm_lib/Frames and Transforms/Rigid Transform  TranslationMethod=Cartesian  TranslationLengthUnit=mm  TranslationStandardAxis=-Y  TranslationStandardOffset=445.61  TranslationCartesianOffset=[-81, -16.3, 0]  TranslationROffset=0  TranslationROffsetUnits=m  TranslationZOffset=0  TranslationZOffsetUnits=m  TranslationThetaOffset=0  TranslationThetaOffsetUnits=deg  RotationMethod=None  RotationAngleUnits=deg  RotationStandardAxis=+Z  RotationAngle=0  RotationArbitraryAxis=[0 0 1]  FollAlignAxisA=+X  BaseAlignAxisA=+Y  FollAlignAxisB=+Y  BaseAlignAxisB=+Z  BlockFunction=simmechanics.library.frames_transforms.rigid_transform
  " Ankle Input Joint" : PMIOPort  Port=1  Side=Right
  Tendon Bearing : PMIOPort  Port=2  Side=Left
  Ball : PMIOPort  Port=3  Side=Left
  Heel : PMIOPort  Port=4  Side=Right
  connections:
  Heel/RConn1 -- To Heel/RConn1
  Ball/RConn1 -- To Ball/RConn1
  To Ball/LConn1 -- To Heel/LConn1 -- To CG/LConn1 -- Shank/RConn1 -- " Ankle Input Joint"/RConn1 -- To Tendon/LConn1
  CG/RConn1 -- To CG/RConn1
  Tendon Bearing/RConn1 -- To Tendon/RConn1

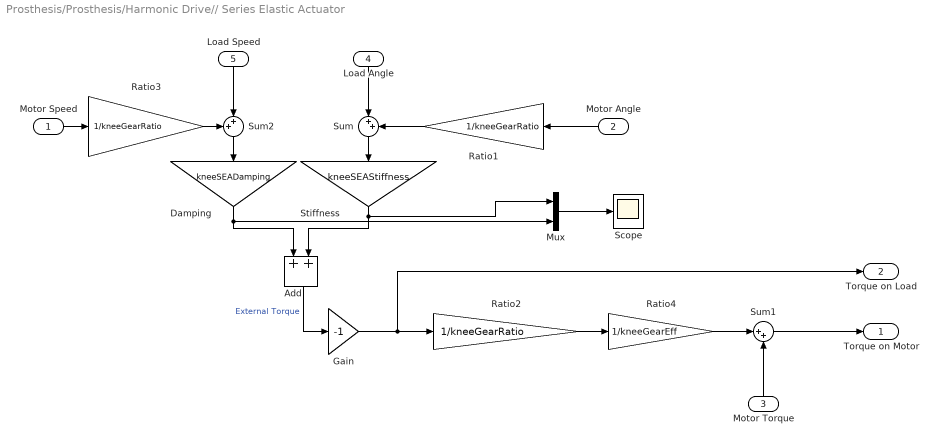
== system Prosthesis/Prosthesis/Harmonic Drive// Series Elastic Actuator ==
  Motor Speed : Inport
  Motor Angle : Inport  Port=2
  Motor Torque : Inport  Port=3
  Load Angle : Inport  Port=4
  Load Speed : Inport  Port=5
  Add : Sum
  Damping : Gain  Gain=kneeSEADamping
  Gain : Gain  Gain=-1
  Mux : Mux  Inputs=2
  Ratio1 : Gain  Gain=1/kneeGearRatio
  Ratio2 : Gain  Gain=1/kneeGearRatio
  Ratio3 : Gain  Gain=1/kneeGearRatio
  Ratio4 : Gain  Gain=1/kneeGearEff
  Scope : Scope
  Stiffness : Gain  Gain=kneeSEAStiffness
  Sum : Sum  Inputs=|++
  Sum1 : Sum  Inputs=|++
  Sum2 : Sum  Inputs=++|
  Torque on Motor : Outport
  " Torque on Load" : Outport  Port=2
  wires:
  Gain/1 -> Ratio2/1, " Torque on Load"/1
  Ratio4/1 -> Sum1/1
  Motor Angle/1 -> Ratio1/1
  Motor Speed/1 -> Ratio3/1
  Sum2/1 -> Damping/1
  Damping/1 -> Mux/2, Add/1
  Sum/1 -> Stiffness/1
  Stiffness/1 -> Mux/1, Add/2
  Sum1/1 -> Torque on Motor/1
  Ratio1/1 -> Sum/2
  Add/1 -> Gain/1  "External Torque"
  Load Angle/1 -> Sum/1
  Ratio2/1 -> Ratio4/1
  Motor Torque/1 -> Sum1/2
  Ratio3/1 -> Sum2/1
  Load Speed/1 -> Sum2/2
  Mux/1 -> Scope/1

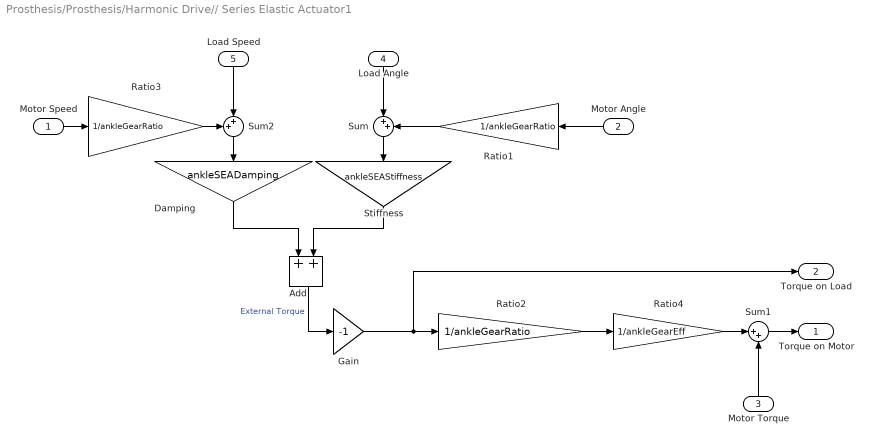
== system Prosthesis/Prosthesis/Harmonic Drive// Series Elastic Actuator1 ==
  Motor Speed : Inport
  Motor Angle : Inport  Port=2
  Motor Torque : Inport  Port=3
  Load Angle : Inport  Port=4
  Load Speed : Inport  Port=5
  Add : Sum
  Damping : Gain  Gain=ankleSEADamping
  Gain : Gain  Gain=-1
  Ratio1 : Gain  Gain=1/ankleGearRatio
  Ratio2 : Gain  Gain=1/ankleGearRatio
  Ratio3 : Gain  Gain=1/ankleGearRatio
  Ratio4 : Gain  Gain=1/ankleGearEff
  Stiffness : Gain  Gain=ankleSEAStiffness
  Sum : Sum  Inputs=|++
  Sum1 : Sum  Inputs=|++
  Sum2 : Sum  Inputs=++|
  Torque on Motor : Outport
  Torque on Load : Outport  Port=2
  wires:
  Ratio4/1 -> Sum1/1
  Motor Angle/1 -> Ratio1/1
  Motor Speed/1 -> Ratio3/1
  Sum2/1 -> Damping/1
  Damping/1 -> Add/1
  Sum/1 -> Stiffness/1
  Stiffness/1 -> Add/2
  Sum1/1 -> Torque on Motor/1
  Ratio1/1 -> Sum/2
  Add/1 -> Gain/1  "External Torque"
  Load Angle/1 -> Sum/1
  Ratio2/1 -> Ratio4/1
  Motor Torque/1 -> Sum1/2
  Ratio3/1 -> Sum2/1
  Load Speed/1 -> Sum2/2
  Gain/1 -> Ratio2/1, Torque on Load/1

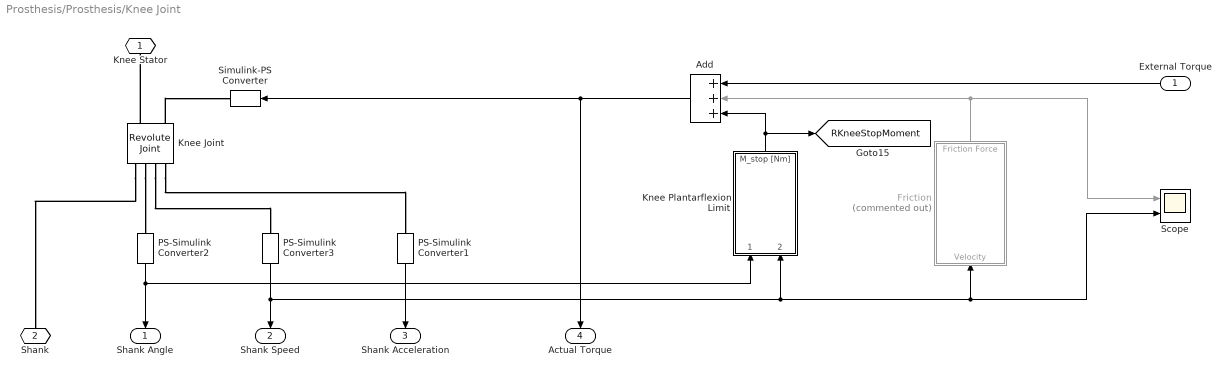
== system Prosthesis/Prosthesis/Knee Joint ==
  External Torque : Inport
  Add : Sum  Inputs=+++
  Friction : Subsystem  Commented=on  mask{Fs=kneeExtStatic, Fc=kneeExtCoulomb, sigma0=dryFrictionStiffness, sigma1=dryFrictionDamping, v_s=dryFrictionVelThresh, Fv=kneeExtDamping}
      mask prompts: Fs "Static Friction"; Fc "Colulomb Friction"; sigma0 "Dry Friction Stiffness"; sigma1 "Dry Friction Damping"; v_s "Velocity Threshold"; Fv "Viscous Friction"
  Knee Joint : sm_lib/Joints/Revolute Joint  SenseConstraintForce=off  SenseConstraintForceX=off  SenseConstraintForceY=off  SenseConstraintForceZ=off  SenseConstraintTorque=off  SenseConstraintTorqueX=off  SenseConstraintTorqueY=off  SenseConstraintTorqueZ=off  SenseTotalForce=off  SenseTotalForceX=off  SenseTotalForceY=off  SenseTotalForceZ=off  SenseTotalTorque=off  SenseTotalTorqueX=off  SenseTotalTorqueY=off  SenseTotalTorqueZ=off  CompositeWrenchDir=FollowerOnBase  CompositeWrenchFrame=BaseFrame  EquilibriumPosition=0  EquilibriumPositionUnits=deg  SpringStiffness=100  SpringStiffnessUnits=N*m/rad  DampingCoefficient=10  DampingCoefficientUnits=N*m/(rad/s)  TorqueActuationMode=InputTorque  MotionActuationMode=ComputedMotion  SensePosition=on  SenseVelocity=on  SenseAcceleration=on  SenseTorqueForce=off  PositionTargetValue=kneeInitialAngle  PositionTargetValueUnits=rad  PositionTargetSpecify=on  PositionTargetPriority=High  VelocityTargetValue=0  VelocityTargetValueUnits=deg/s  VelocityTargetSpecify=off  VelocityTargetPriority=High  BlockFunction=simmechanics.library.joints.revolute_joint
  Knee Plantarflexion Limit : Subsystem  mask{phiUpLimit=0, ext=1, c_jointstop=kneeCJointstop, w_max_jointstop=kneeWMaxJointstop}
      mask prompts: phiUpLimit "Upper Limit [rad]"; ext "Extension values are positive or negative?"; c_jointstop "Stiffness"; w_max_jointstop "Max retraction speed"
      mask help:
      | This block implements a hard joint limit that will prevent the joint from extending past the specified upper limit.
      |
      | Used for the knee and hip joints.
  PS-Simulink Converter1 : nesl_utility/PS-Simulink Converter  PhysicalDomain=network_engine_domain  SubClassName=ps_output  LeftPortType=input  RightPortType=output  PseudoPeriodic=off  Frequencies=[]  Unit=rad/s^2  AffineConversion=off
  PS-Simulink Converter2 : nesl_utility/PS-Simulink Converter  PhysicalDomain=network_engine_domain  SubClassName=ps_output  LeftPortType=input  RightPortType=output  PseudoPeriodic=off  Frequencies=[]  Unit=rad  AffineConversion=off
  PS-Simulink Converter3 : nesl_utility/PS-Simulink Converter  PhysicalDomain=network_engine_domain  SubClassName=ps_output  LeftPortType=input  RightPortType=output  PseudoPeriodic=off  Frequencies=[]  Unit=rad/s  AffineConversion=off
  Scope : Scope  NumInputPorts=2
      settings: TimeRange=5  YMin=-0.5~-4  YMax=0.5~5  SaveName=ScopeData4
  Simulink-PS Converter : nesl_utility/Simulink-PS Converter  PhysicalDomain=network_engine_domain  SubClassName=ps_input  LeftPortType=input  RightPortType=output  PseudoPeriodic=off  Frequencies=[]  NoiseDistribution=none  NoiseParameters=[]  Unit=N*m  AffineConversion=off  InputFiltering=off  SimscapeFilterOrder=1  InputFilterTimeConstant=0.001  UdotUserProvided=1
  Knee Stator : PMIOPort  Port=1  Side=Right
  Shank : PMIOPort  Port=2  Side=Left
  Shank Angle : Outport
  Shank Speed : Outport  Port=2
  Shank Acceleration : Outport  Port=3
  Actual Torque : Outport  Port=4
  tag scope: RKneeStopMoment=global
  wires:
  Friction/1(Friction Force) -> Scope/1, Add/2
  External Torque/1 -> Add/1
  Add/1 -> Simulink-PS Converter/1, Actual Torque/1
  PS-Simulink Converter1/1 -> Shank Acceleration/1
  PS-Simulink Converter3/1 -> Shank Speed/1, Friction/1(Velocity), Scope/2, Knee Plantarflexion Limit/2(dphi [rad/s])
  PS-Simulink Converter2/1 -> Shank Angle/1, Knee Plantarflexion Limit/1(phi [rad])
  Knee Plantarflexion Limit/1(M_stop [Nm]) -> [RKneeStopMoment], Add/3
  connections:
  Knee Joint/RConn4 -- PS-Simulink Converter1/LConn1
  Knee Joint/LConn2 -- Simulink-PS Converter/RConn1
  Knee Joint/RConn2 -- PS-Simulink Converter2/LConn1
  Knee Joint/RConn3 -- PS-Simulink Converter3/LConn1
  Knee Joint/RConn1 -- Shank/RConn1
  Knee Joint/LConn1 -- Knee Stator/RConn1

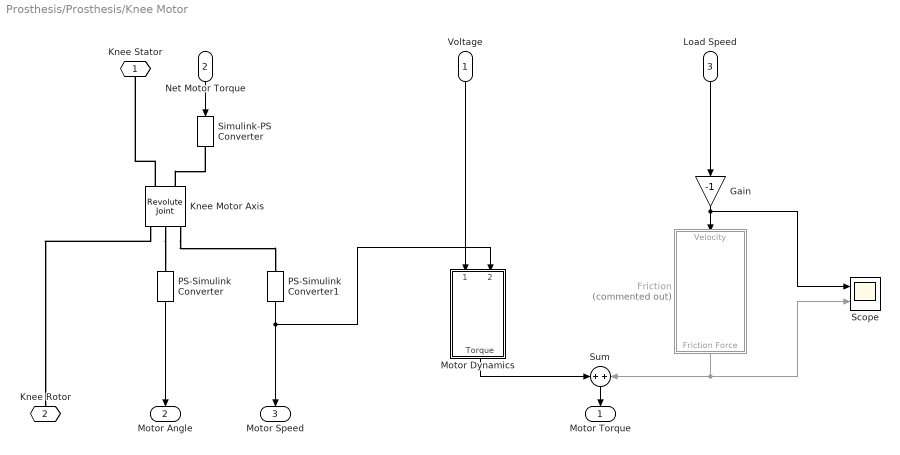
== system Prosthesis/Prosthesis/Knee Motor ==
  Voltage : Inport
  Net Motor Torque : Inport  Port=2
  Load Speed : Inport  Port=3
  Friction : Subsystem  Commented=on  mask{Fs=kneeIntStatic, Fc=kneeIntCoulomb, sigma0=dryFrictionStiffness, sigma1=dryFrictionDamping, v_s=dryFrictionVelThresh, Fv=kneeIntDamping}
      mask prompts: Fs "Static Friction"; Fc "Colulomb Friction"; sigma0 "Dry Friction Stiffness"; sigma1 "Dry Friction Damping"; v_s "Velocity Threshold"; Fv "Viscous Friction"
  Gain : Gain  Gain=-1
  Knee Motor Axis : sm_lib/Joints/Revolute Joint  SenseConstraintForce=off  SenseConstraintForceX=off  SenseConstraintForceY=off  SenseConstraintForceZ=off  SenseConstraintTorque=off  SenseConstraintTorqueX=off  SenseConstraintTorqueY=off  SenseConstraintTorqueZ=off  SenseTotalForce=off  SenseTotalForceX=off  SenseTotalForceY=off  SenseTotalForceZ=off  SenseTotalTorque=off  SenseTotalTorqueX=off  SenseTotalTorqueY=off  SenseTotalTorqueZ=off  CompositeWrenchDir=FollowerOnBase  CompositeWrenchFrame=BaseFrame  EquilibriumPosition=0  EquilibriumPositionUnits=deg  SpringStiffness=0  SpringStiffnessUnits=N*m/deg  DampingCoefficient=0  DampingCoefficientUnits=N*m/(deg/s)  TorqueActuationMode=InputTorque  MotionActuationMode=ComputedMotion  SensePosition=on  SenseVelocity=on  SenseAcceleration=off  SenseTorqueForce=off  PositionTargetValue=-kneeInitialAngle*kneeGearRatio  PositionTargetValueUnits=rad  PositionTargetSpecify=on  PositionTargetPriority=High  VelocityTargetValue=0  VelocityTargetValueUnits=deg/s  VelocityTargetSpecify=off  VelocityTargetPriority=High  BlockFunction=simmechanics.library.joints.revolute_joint
  Motor Dynamics : Subsystem
  PS-Simulink Converter : nesl_utility/PS-Simulink Converter  PhysicalDomain=network_engine_domain  SubClassName=ps_output  LeftPortType=input  RightPortType=output  PseudoPeriodic=off  Frequencies=[]  Unit=rad  AffineConversion=off
  PS-Simulink Converter1 : nesl_utility/PS-Simulink Converter  PhysicalDomain=network_engine_domain  SubClassName=ps_output  LeftPortType=input  RightPortType=output  PseudoPeriodic=off  Frequencies=[]  Unit=rad/s  AffineConversion=off
  Scope : Scope  NumInputPorts=2
      settings: TimeRange=5  YMin=-5~-0.2  YMax=4~0.2
  Simulink-PS Converter : nesl_utility/Simulink-PS Converter  PhysicalDomain=network_engine_domain  SubClassName=ps_input  LeftPortType=input  RightPortType=output  PseudoPeriodic=off  Frequencies=[]  NoiseDistribution=none  NoiseParameters=[]  Unit=N*m  AffineConversion=off  InputFiltering=off  SimscapeFilterOrder=1  InputFilterTimeConstant=0.001  UdotUserProvided=1
  Sum : Sum  Inputs=+|+
  Knee Stator : PMIOPort  Port=1  Side=Right
  Knee Rotor : PMIOPort  Port=2  Side=Left
  Motor Torque : Outport
  Motor Angle : Outport  Port=2
  Motor Speed : Outport  Port=3
  wires:
  Net Motor Torque/1 -> Simulink-PS Converter/1
  Gain/1 -> Scope/1, Friction/1(Velocity)
  Load Speed/1 -> Gain/1
  Friction/1(Friction Force) -> Scope/2, Sum/2
  Motor Dynamics/1(Torque) -> Sum/1
  Sum/1 -> Motor Torque/1
  PS-Simulink Converter1/1 -> Motor Speed/1, Motor Dynamics/2(Speed)
  PS-Simulink Converter/1 -> Motor Angle/1
  Voltage/1 -> Motor Dynamics/1(Voltage)
  connections:
  Knee Motor Axis/RConn1 -- Knee Rotor/RConn1
  Knee Motor Axis/LConn2 -- Simulink-PS Converter/RConn1
  Knee Motor Axis/RConn3 -- PS-Simulink Converter1/LConn1
  Knee Motor Axis/RConn2 -- PS-Simulink Converter/LConn1
  Knee Motor Axis/LConn1 -- Knee Stator/RConn1
